simulink model "ADCS_MIL"  (R2024a)
settings: Solver=FixedStepAuto  StartTime=0.0  StopTime=6000  RelTol=1e-3
undefined symbols (not defined in the file or in its folder): agh, attitude, Cd, dgh, Eearth, epoch, Esun, Jsc, juliandate, k_Bdot, Kd1, Kd2, Kd3, km, Kp1, Kp2, Kp3, m, m_disturb, MTQ_Swithces, NoiseStd, s, satellite, signQuat, simulator, Surf_areas, Surf_dist, Surf_normals, Surf_reflectivity, WMM2020
libraries: sharedtransform x18, aerolibconvert2 x12, SepehrMILLib x11, simulink_extras x8, aerolibsatdyn x5, aerolibutil x5, sharedutil x3, vrlib x3, aerolibtransform2 x3, aerolibgravity2 x3, matrix_library x2
(part 3 of 3)

== system ADCS_MIL/Sensors/Sun Sensor Model ==
  Eclipse : Inport
  q[ICRFtoBody] : Inport  Port=2
  SunPos[ICRF] : Inport  Port=3
  Cartesian to Spherical2 : simulink_extras/Transformations/Cartesian to Spherical
  Demux4 : Demux  Outputs=3
  Demux5 : Demux  Outputs=2
  Eclipse=1 : Constant  Value=0
  Mux2 : Mux  Inputs=3
  Noise_Phi1 : RandomNumber  SampleTime=0.1
  Noise_Theta1 : RandomNumber  SampleTime=0.1
  Pulse Generator1 : DiscretePulseGenerator  Period=10  PulseWidth=5
  Quaternion Rotation1 : aerolibutil/Quaternion Rotation
  Spherical to Cartesian2 : simulink_extras/Transformations/Spherical to Cartesian
  Sum10 : Sum  Inputs=+++
  Sum11 : Sum  Inputs=+++
  SunBias : Constant  Value=[0 0]
  Switch : Switch  Criteria=u2 > Threshold  SaturateOnIntegerOverflow=off  InputSameDT=off
  Switch2 : Switch  Criteria=u2 > Threshold  SaturateOnIntegerOverflow=off  InputSameDT=off
  Zero-Order Hold2 : ZeroOrderHold  SampleTime=-1
  Zero-Order Hold3 : ZeroOrderHold  SampleTime=-1
  SunPos_Sensed(Body) : Outport
  wires:
  Switch2/1 -> SunPos_Sensed(Body)/1
  Noise_Theta1/1 -> Sum10/3
  Spherical to Cartesian2/3 -> Mux2/3
  Demux4/1 -> Cartesian to Spherical2/1
  Spherical to Cartesian2/2 -> Mux2/2
  Demux5/1 -> Sum10/1
  Zero-Order Hold2/1 -> Switch2/1
  Cartesian to Spherical2/1 -> Spherical to Cartesian2/1
  Demux4/2 -> Cartesian to Spherical2/2
  Eclipse=1/1 -> Switch/1
  Spherical to Cartesian2/1 -> Mux2/1
  Mux2/1 -> Switch/3
  Demux5/2 -> Sum11/1
  Sum10/1 -> Spherical to Cartesian2/2
  Sum11/1 -> Spherical to Cartesian2/3
  Cartesian to Spherical2/2 -> Sum10/2
  Noise_Phi1/1 -> Sum11/3
  Demux4/3 -> Cartesian to Spherical2/3
  Pulse Generator1/1 -> Switch2/2
  SunPos[ICRF]/1 -> Quaternion Rotation1/2
  Eclipse/1 -> Switch/2
  Zero-Order Hold3/1 -> Switch2/3
  Switch/1 -> Zero-Order Hold2/1, Zero-Order Hold3/1
  Cartesian to Spherical2/3 -> Sum11/2
  Quaternion Rotation1/1 -> Demux4/1  "SunPos[Body]"
  SunBias/1 -> Demux5/1
  q[ICRFtoBody]/1 -> Quaternion Rotation1/1

== system ADCS_MIL/Attitude Controlgg/On.Nadir_Pointing/Nadir Pointing/PD Controller ==
  Omega(Body) : Inport
  B(Body) : Inport  Port=2
  q_Error : Inport  Port=3
  Kp : Inport  Port=4
  Kd : Inport  Port=5
  MATLAB Function : MATLAB Function  TreatAsAtomicUnit=on
  m_Command : Outport
  wires:
  MATLAB Function/1(m_Command) -> m_Command/1
  q_Error/1 -> MATLAB Function/1(q_Error)
  Omega(Body)/1 -> MATLAB Function/2(omega_Body)
  Kp/1 -> MATLAB Function/3(Kp)
  Kd/1 -> MATLAB Function/4(Kd)
  B(Body)/1 -> MATLAB Function/5(B_body)

== system ADCS_MIL/Attitude Controlgg/On.Nadir_Pointing/Nadir Pointing/q_Desired Propagator ==
  Ephemeris : Inport
  Attitude Profile (Nadir Pointing) : aerolibsatdyn/Attitude Profile (Nadir Pointing)  outputError=on  outputFinalAttitude=off  portFrame=ICRF  pointingMode=Point at nadir  celestialTarget=Sun  tunablePointing=off  primaryAlignmentSrc=Dialog  primaryAlignment=[0 0 1]  secondaryAlignmentSrc=Dialog  secondaryAlignment=[1 0 0]  constraintFrame=ICRF  primaryConstraintSrc=Dialog  primaryConstraint=[1 0 0]  secondaryConstraintSrc=Dialog  secondaryConstraint=[0 1 0]
  Bus Selector : BusSelector  OutputSignals=X_ICRF,V_ICRF
  MATLAB Function : MATLAB Function  TreatAsAtomicUnit=on
  q_Desired : Outport
  wires:
  Ephemeris/1 -> Bus Selector/1
  Bus Selector/2 -> MATLAB Function/2(v_sat_ICRF)  "<V_ICRF>"
  Bus Selector/1 -> MATLAB Function/1(r_sat_ICRF)  "<X_ICRF>"
  MATLAB Function/1(q_Desired) -> q_Desired/1

== system ADCS_MIL/Attitude Controlgg/On.Nadir_Pointing/Nadir Pointing/q_error Calculator ==
  q_Desired : Inport
  q_Real : Inport  Port=2
  MATLAB Function : MATLAB Function  TreatAsAtomicUnit=on
  q_error : Outport
  wires:
  MATLAB Function/1(q_Error) -> q_error/1
  q_Desired/1 -> MATLAB Function/1(q_Real)
  q_Real/1 -> MATLAB Function/2(q_Desired)

== stateflow chart ADCS_MIL/Attitude Controlgg ==
  state On
    state Detumbling
    state Transition
      entry: Sys_Mode;
    state Nadir_Pointing
    state Sun_Pointing
    Transition -> Detumbling [order 3] : [Sys_Mode == 3]
    (default) -> Transition
    Transition -> Sun_Pointing [order 2] : [NavMode == 2]
        | {ControlMode = 2;}
    Sun_Pointing -> Transition : [NavMode == 1]
        | {ControlMode = 1;}
    Transition -> Nadir_Pointing [order 1] : [NavMode == 1]
        | {ControlMode = 2;}
    Nadir_Pointing -> Transition : [NavMode == 2]
        | {ControlMode = 1;}
  state Off
  (default) -> Off
  Off -> On : [NavMode ~= 0]
      | {ControlMode = 1;}
  On -> Off : [NavMode == 0]
      | {ControlMode = 0;}
  data: sf_internal_action_state_placeholder_data local double size=1 =0; sf_internal_action_state_placeholder_data local double size=1 =0; sf_internal_action_state_placeholder_data local double size=1 =0; sf_internal_action_state_placeholder_data local double size=1 =0; System_Mode input

== matlab function ADCS_MIL/External Disturbance Torque/Magnetic/Att_req_inert1 ==
  data: dgh input; agh input; R input; Bn output; RA_earth_rot input
function Bn = magn_field(dgh,agh,R,RA_earth_rot)
%MAGN_FIELD finds magnetic field values using IGRF13 model
Sphc = car2spher(R);
%[Right accencion [rad], declination [rad], radius [whatever]]
Sphc(1) = Sphc(1)-RA_earth_rot;
B1 = magfd(2020,2,Sphc(3)/1000,Sphc(2),Sphc(1),dgh,agh).*[-1 1 -1]';
%B[colat,azimut,radial]
Bn = [(B1(3)*cos(Sphc(2))+B1(1)*sin(Sphc(2)))*cos(Sphc(1))-B1(2)*sin(Sphc(1));...
    (B1(3)*cos(Sphc(2))+B1(1)*sin(Sphc(2)))*sin(Sphc(1))+B1(2)*cos(Sphc(1));...
    B1(3)*sin(Sphc(2))-B1(1)*cos(Sphc(2))];

== matlab function ADCS_MIL/Attitude Controlgg/On.Nadir_Pointing/Nadir Pointing/PD Controller/MATLAB Function ==
  data: q_Error input; m_Command output; omega_Body input; Kp input; Kd input; B_body input
function m_Command = compute_Magnetic_Dipole_Command(q_Error, omega_Body, Kp, Kd, B_body)
    % This function computes the magnetic dipole command for each axis
    % in the body frame to achieve nadir pointing.
    %
    % Inputs:
    %   q_Error  - [4x1] error quaternion representing attitude error [q0, q1, q2, q3]
    %   omega_B  - [3x1] angular velocity vector in body frame (rad/s)
    %   Kp       - Proportional gain for attitude error
    %   Kd       - Derivative gain for angular velocity damping
    %   B_body   - [3x1] magnetic field vector in body frame (T)
    %
    % Output:
    %   m_Command - [3x1] magnetic dipole command vector in body frame (A*m^2)

    % Check input dimensions
    if length(q_Error) ~= 4 || length(omega_Body) ~= 3 || length(B_body) ~= 3
        error('q_Error must be 4x1, omega_B and B_body must be 3x1 vectors.');
    end
    
    % Calculate proportional term using quaternion error (vector part only)
    q_vec = q_Error(2:4); % Vector part of quaternion error [q1, q2, q3]
    p_term = -Kp * q_vec; % Negative sign to drive error to zero
    
    % Calculate derivative term using angular velocity
    d_term = -Kd * omega_Body;
    
    % Control torque vector (u) in body frame
    u = p_term + d_term;
    
    % Calculate magnetic dipole command m = u x B / ||B||^2
    B_norm_squared = norm(B_body)^2;
    
    if B_norm_squared < 1e-10 % Prevent division by very small numbers
        warning('Magnetic field vector magnitude is too small. Setting m_Command to zero.');
        m_Command = [0; 0; 0];
    else
        m_Command = cross(u, B_body) / B_norm_squared;
    end
end

== matlab function ADCS_MIL/External Disturbance Torque/Drag/MATLAB Function ==
  data: Rearth input; Vearth input; M_drag output; Abn input; Surf_norms input; Surf_areas input; Surf_dist input; Cd input
function M_drag = Drag_torque(Rearth,Vearth,Abn,Surf_norms,Surf_areas,Surf_dist,Cd)
%DRAG_TORQUE finds torque due to aerodynamic drag
w_earth = [0 0 0.000072921]';%[rad/s] earth rotation
v_rel = Vearth-cross(w_earth,Rearth);%[m/s] relative velocity
dens = 3.614e-14*exp(-((norm(Rearth)*1e-3-6375)-700)/88.667);%[kg/m3] interpolation
vrb = Abn*v_rel;
vrbabs = norm(vrb);
vrbv = vrb/vrbabs;
tmp1 = ones(3,6);
tmp2 = dot(Surf_norms,bsxfun(@times, tmp1,vrbv));
Across = Surf_areas'.*tmp2;
F = -1/2*dens*Cd*vrbabs^2*bsxfun(@times,vrbv,Across);%[N]
tmp3 = bsxfun(@times,[1 1 1]',tmp2>0);
M_drag = -sum(cross(Surf_dist,F).*tmp3,2);%[Nm]

== matlab function ADCS_MIL/External Disturbance Torque/Radiation Pressure/MATLAB Function1 ==
  data: R input; M_srp output; Abn input; Surf_norms input; Surf_areas input; Surf_reflec input; Surf_dist input; E input
function M_srp = Albedo(R,Abn,Surf_norms,Surf_areas,Surf_reflec,Surf_dist,E)
%ALBEDO finds torque doe to Earth albedo radiation pressure
Sb = Abn*(-R/norm(R));
c = 299792458;%speed of light m/s
P = E/c;
tmp1=ones(3,6);
tmp2=dot(bsxfun(@times, tmp1,Sb),Surf_norms);

% F = -P*Surf_areas'.*tmp2.*((1-Surf_reflec').*Sb+...
%     (2*Surf_reflec'.*tmp2+2/3*Surf_reflec').*Surf_normals);

one = -P*bsxfun(@times,Surf_areas',tmp2);
two = bsxfun(@times,(1-Surf_reflec'),Sb);
three = 2*bsxfun(@times,Surf_reflec',tmp2);
four = bsxfun(@times,(three+2/3*Surf_reflec'),Surf_norms);
F = bsxfun(@times,one,(two+four));
%M_srp=[0 0 0]';
M_srp = sum(bsxfun(@times,cross(Surf_dist,F),(tmp2>0)),2);

== matlab function ADCS_MIL/External Disturbance Torque/Gravitional/MATLAB Function ==
  data: Rearth input; Vearth input; Abn input; J input; M_grav output
function M_grav = Grav(Rearth,Vearth,Abn,J)
%GRAV calculates torque due to gravity
Mue = 398600.4418e3;%[km3/s2)]Earth gravity parameter
R1 = Rearth/norm(Rearth);
V1 = Vearth/norm(Vearth);
Aln = [R1 V1 cross(R1,V1)];
Abl = Abn/Aln;

M_grav = 3*Mue/norm(Rearth)^3*[(J(3)-J(2))*Abl(3,1)*Abl(2,1);...
                            (J(1)-J(3))*Abl(1,1)*Abl(3,1);...
                            (J(2)-J(1))*Abl(1,1)*Abl(2,1)];

== matlab function ADCS_MIL/External Disturbance Torque/Absolute values ==
  data: s1 input; st output; s2 input; s3 input; s4 input
function st = absolutes(s1,s2,s3,s4)
%calculate absolute disurbance values
st = sqrt(sum([s1 s2 s3 s4].^2,1));

== matlab function ADCS_MIL/Attitude Controlgg/On.Nadir_Pointing/Nadir Pointing/q_Desired Propagator/MATLAB Function ==
  data: r_sat_ICRF input; q_Desired output; v_sat_ICRF input
function q_Desired = compute_desired_quaternion(r_sat_ICRF, v_sat_ICRF)
    % Inputs:
    % r_sat_ECI - Satellite position in ECI(ICRF) frame (3x1 vector)
    % v_sat_ECI - Satellite velocity in ECI(ICRF) frame (3x1 vector)
    
    % Step 1: Compute the nadir vector in ECI(ICRF) frame
    r_nadir_ECI = -r_sat_ICRF;
    Z_LVLH = r_nadir_ECI / norm(r_nadir_ECI); % Normalized nadir direction
    
    % Step 2: Compute the LVLH Y-axis (orbit normal)
    Y_LVLH = cross(r_nadir_ECI, v_sat_ICRF);
    Y_LVLH = Y_LVLH / norm(Y_LVLH); % Normalize orbit normal
    
    % Step 3: Compute the LVLH X-axis (along velocity direction)
    X_LVLH = cross(Y_LVLH, Z_LVLH); % Right-hand rule
    
    % Step 4: Construct the rotation matrix from ECI to LVLH
    R_ECI_LVLH = [X_LVLH, Y_LVLH, Z_LVLH];
    
    % Step 5: Convert rotation matrix to quaternion
    q_Desired = rotm2quat(R_ECI_LVLH); % Desired quaternion for nadir pointing
end

== matlab function ADCS_MIL/Attitude Controlgg/On.Nadir_Pointing/Nadir Pointing/q_error Calculator/MATLAB Function ==
  data: q_Real input; q_Error output; q_Desired input
function q_Error = compute_Error_Quaternion(q_Real, q_Desired)
    % This function computes the error quaternion for Nadir pointing
    % Inputs:
    %   q_Real - [4x1] vector, the actual (real) quaternion [q0, q1, q2, q3]
    %   q_Desired - [4x1] vector, the desired quaternion [q0, q1, q2, q3]
    % Output:
    %   q_Error - [4x1] vector, the error quaternion [q0, q1, q2, q3]

    % Check input dimensions
    if length(q_Real) ~= 4 || length(q_Desired) ~= 4
        error('Both q_Real and q_Desired must be 4-element vectors.');
    end

    % Normalize input quaternions to ensure they are unit quaternions
    q_Real = q_Real / norm(q_Real);
    q_Desired = q_Desired / norm(q_Desired);

    % Conjugate of the desired quaternion
    q_Desired_conj = [q_Desired(1); -q_Desired(2:4)];

    % Compute the error quaternion using quaternion multiplication
    q_Error = [
        q_Desired_conj(1) * q_Real(1) - q_Desired_conj(2) * q_Real(2) - q_Desired_conj(3) * q_Real(3) - q_Desired_conj(4) * q_Real(4);
        q_Desired_conj(1) * q_Real(2) + q_Desired_conj(2) * q_Real(1) + q_Desired_conj(3) * q_Real(4) - q_Desired_conj(4) * q_Real(3);
        q_Desired_conj(1) * q_Real(3) - q_Desired_conj(2) * q_Real(4) + q_Desired_conj(3) * q_Real(1) + q_Desired_conj(4) * q_Real(2);
        q_Desired_conj(1) * q_Real(4) + q_Desired_conj(2) * q_Real(3) - q_Desired_conj(3) * q_Real(2) + q_Desired_conj(4) * q_Real(1)
    ];

    % Normalize the error quaternion to ensure it's a unit quaternion
    q_Error = q_Error / norm(q_Error);
end

== stateflow chart ADCS_MIL/Attitude Control Algorithms ==
  state On
    state Detumbling
    state Transition
      entry: Sys_Mode;
    state Nadir_Pointing
    Transition -> Detumbling [order 2] : [Sys_Mode == 2]
    (default) -> Transition
    Transition -> Nadir_Pointing [order 1] : [Sys_Mode == 4 || Sys_Mode == 7 || Sys_Mode == 9]
  state Off
  (default) -> Off
  Off -> On
  On -> Off
  data: sf_internal_action_state_placeholder_data local double size=1 =0; sf_internal_action_state_placeholder_data local double size=1 =0; sf_internal_action_state_placeholder_data local double size=1 =0; Sys_Mode input

== matlab function ADCS_MIL/External Disturbance Torque/Radiation Pressure/MATLAB Function ==
  data: Rsun input; M_srp output; Abn input; Surf_norms input; Surf_areas input; Surf_reflec input; Surf_dist input; Esun input
function M_srp = SRP(Rsun,Abn,Surf_norms,Surf_areas,Surf_reflec,Surf_dist,Esun)
%SRP finds torque due to SRP
Sb = Abn*(-Rsun/norm(Rsun));
c = 299792458;%[m/s] speed of light
P = Esun/c;%[Pa] Pressure
tmp1=ones(3,6);
tmp2=dot(bsxfun(@times, tmp1,Sb),Surf_norms);

% F = -P*Surf_areas'.*tmp2.*((1-Surf_reflec').*Sb+...
%     (2*Surf_reflec'.*tmp2+2/3*Surf_reflec').*Surf_normals);

one = -P*bsxfun(@times,Surf_areas',tmp2);
two = bsxfun(@times,(1-Surf_reflec'),Sb);
three = 2*bsxfun(@times,Surf_reflec',tmp2);
four = bsxfun(@times,(three+2/3*Surf_reflec'),Surf_norms);
F = bsxfun(@times,one,(two+four));%[N] forces acting
M_srp = sum(bsxfun(@times,cross(Surf_dist,F),(tmp2>0)),2);%[Nm] Torque

== matlab function ADCS_MIL/External Disturbance Torque/Magnetic/Magnetic Disturbance Torques Calculator ==
  data: m_residual input; T_mag_disturb output; B_earth input
function T_mag_disturb = computeMagneticDisturbanceTorque(m_residual, B_earth)
    % Inputs:
    %   m_residual - Residual magnetic moment vector [3x1] in the satellite's body frame (Am^2)
    %   B_earth    - Earth's magnetic field vector [3x1] in the satellite's body frame (T)
    %
    % Output:
    %   T_mag_disturb - Magnetic disturbance torque [3x1] in the satellite's body frame (Nm)

    % Validate inputs
    if length(m_residual) ~= 3 || length(B_earth) ~= 3
        error('Both m_residual and B_earth must be 3-dimensional vectors.');
    end

    % Compute the magnetic disturbance torque
    T_mag_disturb = cross(m_residual, B_earth);
end

== matlab function ADCS_MIL/Orbit Eclipse Calculator/MATLAB Function1 ==
  data: Alpha input; Eclipse output
function Eclipse = AlphaToEclipse(Alpha)
if Alpha < 1.57075 && Alpha >= 0
    Eclipse = 0;
else
    Eclipse = 1;
end

== matlab function ADCS_MIL/Attitude Determination and Estimation Algorithms/MATLAB Function1 ==
  data: SunPos_ECI input; quat_TRIAD output; MagField_ECI input; SunPos_Body input; MagField_Body input; CovarianceMatrix output; RotationMatrix output; NoiseStd input; signQuat input
function [quat_TRIAD, CovarianceMatrix, RotationMatrix] = TRIAD(SunPos_ECI, MagField_ECI, SunPos_Body, MagField_Body, NoiseStd, signQuat)
% TRIAD Algorithm for Attitude Determination
% Inputs:
% - SunPos_ECI: Sun position vector in the inertial frame (ECI)
% - MagField_ECI: Magnetic field vector in the inertial frame (ECI)
% - SunPos_Body: Sun position vector in the body (spacecraft) frame
% - MagField_Body: Magnetic field vector in the body (spacecraft) frame
% - NoiseStd: [sigma1, sigma2] standard deviations of measurement noise
% - signQuat: sign parameter for quaternion calculation (e.g., ±1)
%
% Outputs:
% - quat_TRIAD: Quaternion representing the body-to-inertial rotation
% - CovarianceMatrix: Covariance matrix for the attitude estimation
% - RotationMatrix: Direction Cosine Matrix (DCM) from body to inertial frame

% Separate the noise standard deviations for more accurate and less accurate measurements
sigma_Sun = NoiseStd(1); % Standard deviation for Sun position measurement
sigma_Mag = NoiseStd(2); % Standard deviation for magnetic field measurement

% Reference Frame TRIAD Vectors (in ECI)
ref1 = SunPos_ECI;    % First vector (higher accuracy) in inertial frame
ref2 = cross(SunPos_ECI, MagField_ECI) / norm(cross(SunPos_ECI, MagField_ECI));
ref3 = cross(SunPos_ECI, ref2);  % Complete orthogonal basis

RefFrameMatrix = [ref1, ref2, ref3]; % TRIAD frame in terms of ECI vectors

% Body Frame TRIAD Vectors (in Spacecraft Frame)
body1 = SunPos_Body;  % First vector (higher accuracy) in body frame
body2 = cross(SunPos_Body, MagField_Body) / norm(cross(SunPos_Body, MagField_Body));
body3 = cross(SunPos_Body, body2); % Complete orthogonal basis

BodyFrameMatrix = [body1, body2, body3]; % TRIAD frame in terms of body vectors

% Estimated Rotation Matrix (DCM) from Body to Inertial Frame
RotationMatrix = RefFrameMatrix * BodyFrameMatrix';
RotationMatrix = transpose(RotationMatrix); % Transpose if convention requires it

% Convert Rotation Matrix to Quaternion
quat_TRIAD = DCMtoQuaternion(RotationMatrix, signQuat);

% Covariance Matrix Calculation for TRIAD
CovarianceMatrix = 0;
% CovarianceMatrix = (sigma_Sun^2 * eye(3)) + ...
%     (((sigma_Mag^2 - sigma_Sun^2) * (body1 * body1')) + ...
%     (sigma_Sun^2 * (dot(body1, body2) * ((body1 * body2') + (body2 * body1'))))) / ...
%     (norm(cross(body1, body2))^2));

end

== matlab function ADCS_MIL/Nadir Pointing Algorithm/PD Controller/MATLAB Function ==
  data: q_Error input; m_Command output; omega_Body input; Kp input; Kd input; B_body input
function m_Command = compute_Magnetic_Dipole_Command(q_Error, omega_Body, Kp, Kd, B_body)
    % This function computes the magnetic dipole command for each axis
    % in the body frame to achieve nadir pointing.
    %
    % Inputs:
    %   q_Error  - [4x1] error quaternion representing attitude error [q0, q1, q2, q3]
    %   omega_B  - [3x1] angular velocity vector in body frame (rad/s)
    %   Kp       - Proportional gain for attitude error
    %   Kd       - Derivative gain for angular velocity damping
    %   B_body   - [3x1] magnetic field vector in body frame (T)
    %
    % Output:
    %   m_Command - [3x1] magnetic dipole command vector in body frame (A*m^2)

    % Check input dimensions
    if length(q_Error) ~= 4 || length(omega_Body) ~= 3 || length(B_body) ~= 3
        error('q_Error must be 4x1, omega_B and B_body must be 3x1 vectors.');
    end
    
    % Calculate proportional term using quaternion error (vector part only)
    q_vec = q_Error(2:4); % Vector part of quaternion error [q1, q2, q3]
    p_term = -Kp * q_vec; % Negative sign to drive error to zero
    
    % Calculate derivative term using angular velocity
    d_term = -Kd * omega_Body;
    
    % Control torque vector (u) in body frame
    u = p_term + d_term;
    
    % Calculate magnetic dipole command m = u x B / ||B||^2
    B_norm_squared = norm(B_body)^2;
    
    if B_norm_squared < 1e-10 % Prevent division by very small numbers
        warning('Magnetic field vector magnitude is too small. Setting m_Command to zero.');
        m_Command = [0; 0; 0];
    else
        m_Command = cross(u, B_body) / B_norm_squared;
    end
end

== matlab function ADCS_MIL/Detumbling Algorithm/MATLAB Function ==
  data: vector input; length output
function length = vector_length(vector)
    length = sqrt(sum(vector.^2));
end

== matlab function ADCS_MIL/Nadir Pointing Algorithm/q_Desired Propagator/MATLAB Function ==
  data: r_sat_ICRF input; q_Desired output; v_sat_ICRF input
function q_Desired = compute_desired_quaternion(r_sat_ICRF, v_sat_ICRF)
    % Inputs:
    % r_sat_ECI - Satellite position in ECI(ICRF) frame (3x1 vector)
    % v_sat_ECI - Satellite velocity in ECI(ICRF) frame (3x1 vector)
    
    % Step 1: Compute the nadir vector in ECI(ICRF) frame
    r_nadir_ECI = -r_sat_ICRF;
    Z_LVLH = r_nadir_ECI / norm(r_nadir_ECI); % Normalized nadir direction
    
    % Step 2: Compute the LVLH Y-axis (orbit normal)
    Y_LVLH = cross(r_nadir_ECI, v_sat_ICRF);
    Y_LVLH = Y_LVLH / norm(Y_LVLH); % Normalize orbit normal
    
    % Step 3: Compute the LVLH X-axis (along velocity direction)
    X_LVLH = cross(Y_LVLH, Z_LVLH); % Right-hand rule
    
    % Step 4: Construct the rotation matrix from ECI to LVLH
    R_ECI_LVLH = [X_LVLH, Y_LVLH, Z_LVLH];
    
    % Step 5: Convert rotation matrix to quaternion
    q_Desired = rotm2quat(R_ECI_LVLH); % Desired quaternion for nadir pointing
end

== matlab function ADCS_MIL/Nadir Pointing Algorithm/q_error Calculator/MATLAB Function ==
  data: q_Real input; q_Error output; q_Desired input
function q_Error = compute_Error_Quaternion(q_Real, q_Desired)
    % This function computes the error quaternion for Nadir pointing
    % Inputs:
    %   q_Real - [4x1] vector, the actual (real) quaternion [q0, q1, q2, q3]
    %   q_Desired - [4x1] vector, the desired quaternion [q0, q1, q2, q3]
    % Output:
    %   q_Error - [4x1] vector, the error quaternion [q0, q1, q2, q3]

    % Check input dimensions
    if length(q_Real) ~= 4 || length(q_Desired) ~= 4
        error('Both q_Real and q_Desired must be 4-element vectors.');
    end

    % Normalize input quaternions to ensure they are unit quaternions
    q_Real = q_Real / norm(q_Real);
    q_Desired = q_Desired / norm(q_Desired);

    % Conjugate of the desired quaternion
    q_Desired_conj = [q_Desired(1); -q_Desired(2:4)];

    % Compute the error quaternion using quaternion multiplication
    q_Error = [
        q_Desired_conj(1) * q_Real(1) - q_Desired_conj(2) * q_Real(2) - q_Desired_conj(3) * q_Real(3) - q_Desired_conj(4) * q_Real(4);
        q_Desired_conj(1) * q_Real(2) + q_Desired_conj(2) * q_Real(1) + q_Desired_conj(3) * q_Real(4) - q_Desired_conj(4) * q_Real(3);
        q_Desired_conj(1) * q_Real(3) - q_Desired_conj(2) * q_Real(4) + q_Desired_conj(3) * q_Real(1) + q_Desired_conj(4) * q_Real(2);
        q_Desired_conj(1) * q_Real(4) + q_Desired_conj(2) * q_Real(3) - q_Desired_conj(3) * q_Real(2) + q_Desired_conj(4) * q_Real(1)
    ];

    % Normalize the error quaternion to ensure it's a unit quaternion
    q_Error = q_Error / norm(q_Error);
end
